simulink library "Orbit"  (R2014b)
settings: Solver=ode45  StartTime=0.0  StopTime=10.0  RelTol=1e-3
undefined symbols (not defined in the file or in its folder): ConfParam
libraries: ECEFtoJ2000 x1, J2000toGeoc x1, Normalization x1
settings Model: Creator=Hp  LastModifiedBy=Hp

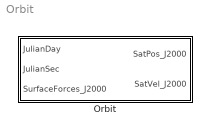
== system Orbit ==
  Orbit : Subsystem

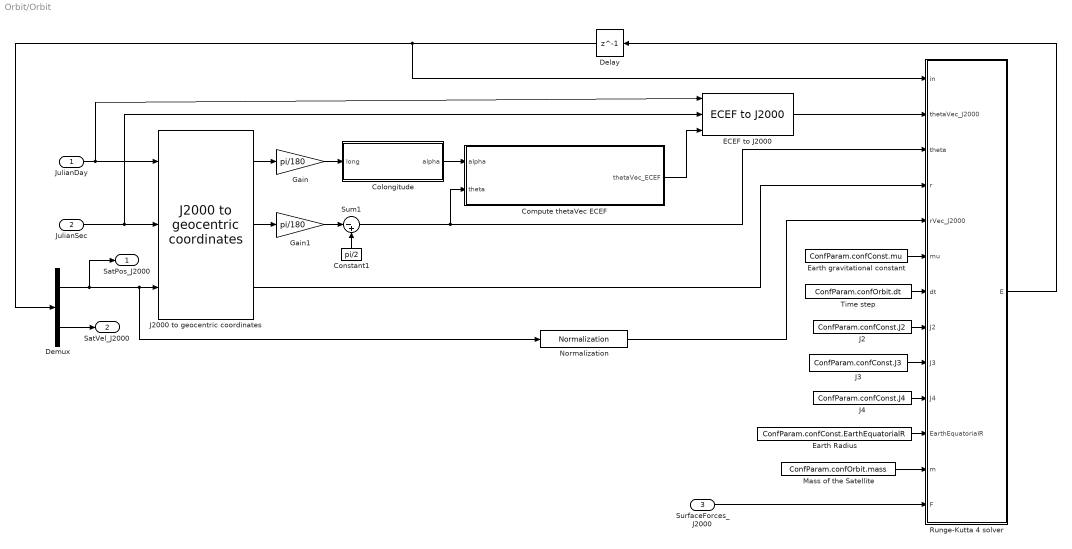
== system Orbit/Orbit ==
  JulianDay : Inport
  JulianSec : Inport  Port=2
  SurfaceForces_J2000 : Inport  Port=3
  Colongitude : MATLAB Function  TreatAsAtomicUnit=on
  Compute thetaVec ECEF : MATLAB Function  TreatAsAtomicUnit=on
  Constant1 : Constant  Value=pi/2
  Delay : Delay  DelayLength=1  InitialCondition=ConfParam.confOrbit.InitOrbit  SampleTime=ConfParam.confOrbit.dt
  Demux : Demux  Outputs=2
  ECEF to J2000 : ECEFtoJ2000/ECEF to J2000
  Earth Radius : Constant  Value=ConfParam.confConst.EarthEquatorialR
  Earth gravitational constant : Constant  Value=ConfParam.confConst.mu
  Gain : Gain  Gain=pi/180
  Gain1 : Gain  Gain=pi/180
  J2 : Constant  Value=ConfParam.confConst.J2
  J2000 to geocentric coordinates : J2000toGeoc/J2000 to geocentric coordinates
  J3 : Constant  Value=ConfParam.confConst.J3
  J4 : Constant  Value=ConfParam.confConst.J4
  Mass of the Satellite : Constant  Value=ConfParam.confOrbit.mass
  Normalization : Normalization/Normalization
  Runge-Kutta 4 solver : MATLAB Function  TreatAsAtomicUnit=on
  Sum1 : Sum  Inputs=|-+
  Time step : Constant  Value=ConfParam.confOrbit.dt
  SatPos_J2000 : Outport
  SatVel_J2000 : Outport  Port=2
  wires:
  Delay/1 -> Demux/1, Runge-Kutta 4 solver/1(in)
  Time step/1 -> Runge-Kutta 4 solver/7(dt)
  Earth gravitational constant/1 -> Runge-Kutta 4 solver/6(mu)
  Runge-Kutta 4 solver/1(E) -> Delay/1
  Demux/2 -> SatVel_J2000/1
  JulianDay/1 -> J2000 to geocentric coordinates/1, ECEF to J2000/1
  JulianSec/1 -> J2000 to geocentric coordinates/2, ECEF to J2000/2
  J2000 to geocentric coordinates/1 -> Gain/1
  J2000 to geocentric coordinates/2 -> Gain1/1
  Gain1/1 -> Sum1/1
  Constant1/1 -> Sum1/2
  Sum1/1 -> Runge-Kutta 4 solver/3(theta), Compute thetaVec ECEF/2(theta)
  Demux/1 -> SatPos_J2000/1, J2000 to geocentric coordinates/3, Normalization/1
  J2000 to geocentric coordinates/3 -> Runge-Kutta 4 solver/4(r)
  J2/1 -> Runge-Kutta 4 solver/8(J2)
  J4/1 -> Runge-Kutta 4 solver/10(J4)
  Earth Radius/1 -> Runge-Kutta 4 solver/11(EarthEquatorialR)
  Compute thetaVec ECEF/1(thetaVec_ECEF) -> ECEF to J2000/3
  ECEF to J2000/1 -> Runge-Kutta 4 solver/2(thetaVec_J2000)
  Normalization/1 -> Runge-Kutta 4 solver/5(rVec_J2000)
  Gain/1 -> Colongitude/1(long)
  Colongitude/1(alpha) -> Compute thetaVec ECEF/1(alpha)
  J3/1 -> Runge-Kutta 4 solver/9(J3)
  Mass of the Satellite/1 -> Runge-Kutta 4 solver/12(m)
  SurfaceForces_J2000/1 -> Runge-Kutta 4 solver/13(F)

== matlab function Orbit/Colongitude ==
  data: long input; alpha output
function alpha = colongitude(long)
    if long<0
        alpha=2*pi+long;
    else
        alpha=long;
    end
end

== matlab function Orbit/Compute thetaVec ECEF ==
  data: alpha input; theta input; thetaVec_ECEF output
function thetaVec_ECEF = ComputeThetaVec(alpha, theta)

    i=[1; 0; 0]; j=[0; 1; 0]; k=[0; 0; 1];
    
    thetaVec_ECEF = cos(theta)*cos(alpha)*i+cos(theta)*sin(alpha)*j-sin(theta)*k;
    
end

== matlab function Orbit/Runge-Kutta 4 solver ==
  data: in input; thetaVec_J2000 input; theta input; r input; rVec_J2000 input; E output; mu input; dt input; J2 input; J3 input; J4 input; EarthEquatorialR input; m input; F input
function E=RK4(in, thetaVec_J2000, theta, r, rVec_J2000, mu, dt, J2, J3, J4, EarthEquatorialR, m, F)
    % Runge-Kutta 4 solver      
    E=in;
    Ei=in;
    
    K1=DifferentialEq(Ei, thetaVec_J2000, theta, rVec_J2000, r, mu, J2, J3, J4, EarthEquatorialR, m, F);
    
    Ei=E+dt/2*K1;
    K2=DifferentialEq(Ei, thetaVec_J2000, theta, rVec_J2000, r, mu, J2, J3, J4, EarthEquatorialR, m, F);
    
    Ei=E+dt/2*K2;
    K3=DifferentialEq(Ei, thetaVec_J2000, theta, rVec_J2000, r, mu, J2, J3, J4, EarthEquatorialR, m, F);
    
    Ei=E+dt*K3;
    K4=DifferentialEq(Ei, thetaVec_J2000, theta, rVec_J2000, r, mu, J2, J3, J4, EarthEquatorialR, m, F);
    
    E=E+dt/6*(K1+2*(K2+K3)+K4);

end
